simulink model "iq_modulation"  (R2014b)
settings: Solver=ode45  StartTime=0.0  StopTime=inf  RelTol=1e-3
libraries: dsparch4 x2
settings Model: Creator=Ben  LastModifiedBy=Ben

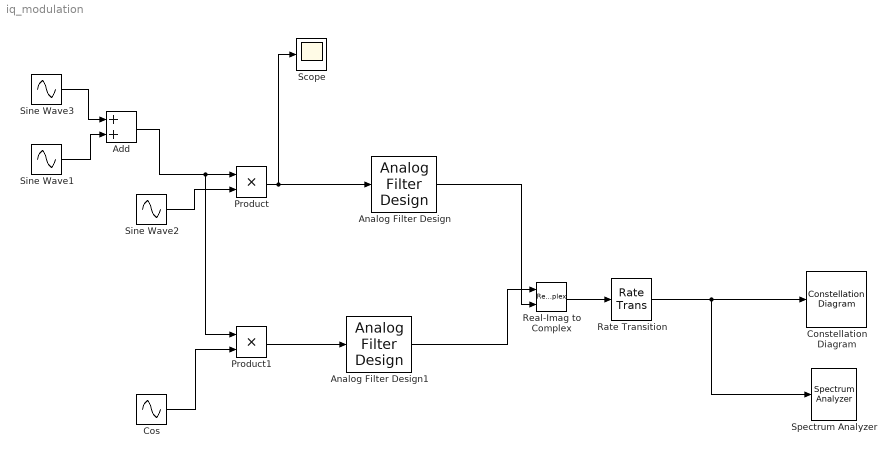
== system iq_modulation ==
  Add : Sum
  Analog Filter Design : dsparch4/Analog Filter Design  method=Butterworth  filttype=Lowpass  N=8  Wlo=2  Whi=80  Rp=2  Rs=40
  Analog Filter Design1 : dsparch4/Analog Filter Design  method=Butterworth  filttype=Lowpass  N=8  Wlo=2  Whi=80  Rp=2  Rs=40
  Constellation Diagram : ConstellationDiagram
  "Cos " : Sin  Frequency=11  Phase=-1*pi/2  SampleTime=0.001
  Product : Product
  Product1 : Product
  Rate Transition : RateTransition  OutPortSampleTime=.1
  Real-Imag to Complex : RealImagToComplex
  Scope : Scope
  Sine Wave1 : Sin  Frequency=12  SampleTime=0.001
  Sine Wave2 : Sin  Frequency=11  SampleTime=0.001
  Sine Wave3 : Sin  Frequency=10  SampleTime=0.001
  Spectrum Analyzer : SpectrumAnalyzer
  wires:
  Add/1 -> Product1/1, Product/1
  Sine Wave2/1 -> Product/2
  "Cos "/1 -> Product1/2
  Product/1 -> Scope/1, Analog Filter Design/1
  Product1/1 -> Analog Filter Design1/1
  Real-Imag to Complex/1 -> Rate Transition/1
  Sine Wave3/1 -> Add/1
  Sine Wave1/1 -> Add/2
  Analog Filter Design/1 -> Real-Imag to Complex/2
  Analog Filter Design1/1 -> Real-Imag to Complex/1
  Rate Transition/1 -> Spectrum Analyzer/1, Constellation Diagram/1
